simulink model "TestGroup_v2"  (R2024b)
settings: Solver=VariableStepAuto  StartTime=0.0  StopTime=45  RelTol=1e-3
model workspace (MAT data in the model file):
  K1 = 1
  K2 = 1
  K3 = 1
values from neighbouring files (symbols this model uses):
  A_altitude = [ ... (first row only)    [STATE_SPACE_CALCULATIONS.m]
  B_altitude = [ ... (first row only)    [STATE_SPACE_CALCULATIONS.m]
  C_altitude = [1, 0, 0]    [STATE_SPACE_CALCULATIONS.m]
  D_altitude = [0]    [STATE_SPACE_CALCULATIONS.m]
  K_altitude = lqr(A_altitude, B_altitude, Q_altitude, R_altitude)    [STATE_SPACE_CALCULATIONS.m]
settings Model: Creator=hazza  LastModifiedBy=hazza

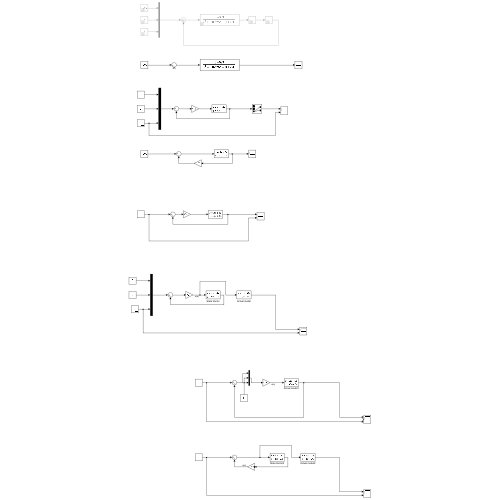
[thumbnail: Simulink's stored preview of the top-level diagram]
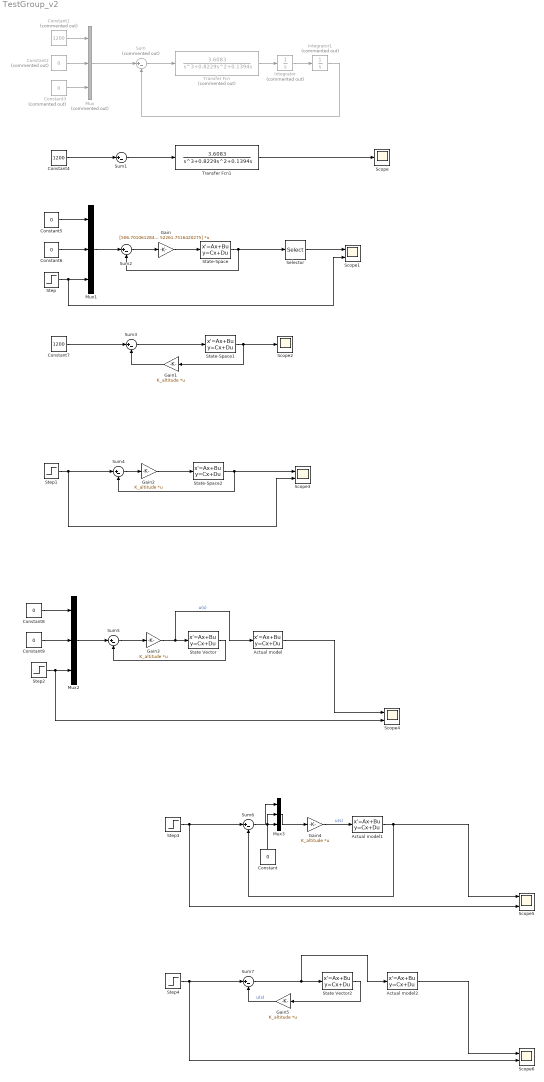
== system TestGroup_v2 ==
  Actual model : StateSpace  A=A_altitude  B=B_altitude  C=C_altitude  D=D_altitude  InitialCondition=[0 0 1200]
  Actual model1 : StateSpace  A=A_altitude  B=B_altitude  C=C_altitude  D=D_altitude  InitialCondition=[0 0 0]
  Actual model2 : StateSpace  A=A_altitude  B=B_altitude  C=C_altitude  D=D_altitude  InitialCondition=[0 0 0]
  Constant{,5..6,8..9} (5 alike) : Constant  Value=0
  Constant1 : Constant  Commented=on  Value=1200
  Constant2 : Constant  Commented=on  Value=0
  Constant3 : Constant  Commented=on  Value=0
  Constant4 : Constant  Value=1200
  Constant7 : Constant  Value=1200
  Gain : Gain  Gain=[506.70106128442 676.986305298063 52261.7516420275]  Multiplication=Matrix(K*u)
  Gain{1..5} (5 alike) : Gain  Gain=K_altitude  Multiplication=Matrix(K*u)
  Integrator : Integrator  Commented=on
  Integrator1 : Integrator  Commented=on
  Mux : Mux  Commented=on  Inputs=3
  Mux1 : Mux  Inputs=3
  Mux2 : Mux  Inputs=3
  Mux3 : Mux  Inputs=3
  Scope : Scope
  Scope{1,3..4,6} (4 alike) : Scope  NumInputPorts=2
  Scope2 : Scope
  Scope5 : Scope  NumInputPorts=3
  Selector : Selector  InputPortWidth=3  IndexOptions=Index vector (dialog)  Indices=[3 3]  OutputSizes=1
  State Vector : StateSpace  A=A_altitude  B=B_altitude  C=[1 0 0; 0 1 0; 0 0 1]  D=[0; 0; 0]  InitialCondition=[0 0 1200]
  State Vector2 : StateSpace  A=A_altitude  B=B_altitude  C=[0 0 1; 0 1 0; 1 0 0]  D=[0; 0; 0]  InitialCondition=[0 0 0]
  State-Space : StateSpace  A=A_altitude  B=B_altitude  C=[1 0 0; 0 1 0; 0 0 1]  D=[0; 0; 0]  InitialCondition=[0, 0, 1000]
  State-Space1 : StateSpace  A=A_altitude  B=B_altitude  C=[1 0 0; 0 1 0; 0 0 1]  D=[0; 0; 0]  InitialCondition=[1200, 0,0 ]
  State-Space2 : StateSpace  A=A_altitude  B=B_altitude  C=[1 0 0; 0 1 0; 0 0 1]  D=[0; 0; 0]  InitialCondition=[0, 0, 1500]
  Step : Step  Time=5  Before=1500  After=1200  SampleTime=0
  Step1 : Step  Time=5  Before=1500  After=1200  SampleTime=0
  Step2 : Step  Time=5  Before=1500  After=1200  SampleTime=0
  Step3 : Step  After=10  SampleTime=0
  Step4 : Step  After=10  SampleTime=0
  Sum : Sum  Commented=on  Inputs=|+-
  Sum{1..7} (7 alike) : Sum  Inputs=|+-
  Transfer Fcn : TransferFcn  Commented=on  Numerator=3.6083  Denominator=[1, 0.8229, 0.1394, 0]
  Transfer Fcn1 : TransferFcn  Numerator=3.6083  Denominator=[1, 0.8229, 0.1394, 0]
  wires:
  Constant4/1 -> Sum1/1
  Transfer Fcn1/1 -> Scope/1
  Constant2/1 -> Mux/2
  Integrator/1 -> Integrator1/1
  Mux/1 -> Sum/1
  Integrator1/1 -> Sum/2
  Constant7/1 -> Sum3/1
  Sum1/1 -> Transfer Fcn1/1
  Mux1/1 -> Sum2/1
  Constant1/1 -> Mux/1
  Sum/1 -> Transfer Fcn/1
  State-Space1/1 -> Gain1/1, Scope2/1
  Gain/1 -> State-Space/1
  Sum3/1 -> State-Space1/1
  Gain1/1 -> Sum3/2
  State-Space/1 -> Sum2/2, Selector/1
  Sum2/1 -> Gain/1
  Constant3/1 -> Mux/3
  Transfer Fcn/1 -> Integrator/1
  Constant5/1 -> Mux1/1
  Constant6/1 -> Mux1/2
  Step/1 -> Scope1/2, Mux1/3
  Step1/1 -> Sum4/1, Scope3/2
  State-Space2/1 -> Sum4/2, Scope3/1
  Sum4/1 -> Gain2/1
  Gain2/1 -> State-Space2/1
  Selector/1 -> Scope1/1
  Step2/1 -> Scope4/2, Mux2/3
  State Vector/1 -> Sum5/2
  Gain3/1 -> Actual model/1, State Vector/1  "u(s)"
  Mux2/1 -> Sum5/1
  Sum5/1 -> Gain3/1
  Constant8/1 -> Mux2/1
  Constant9/1 -> Mux2/2
  Actual model/1 -> Scope4/1
  Step3/1 -> Scope5/3, Sum6/1
  Actual model1/1 -> Sum6/2, Scope5/1
  Step4/1 -> Scope6/2, Sum7/1
  Sum7/1 -> Actual model2/1, State Vector2/1
  State Vector2/1 -> Gain5/1
  Gain5/1 -> Sum7/2  "u(s)"
  Actual model2/1 -> Scope6/1
  Gain4/1 -> Actual model1/1  "u(s)"
  Mux3/1 -> Gain4/1
  Sum6/1 -> Mux3/1
  Constant/1 -> Mux3/2, Mux3/3
